simulink model "spectra_signals_new_2020b"  (R2020b)
settings: Solver=ode45  StartTime=0.0  StopTime=4.4  RelTol=1e-3  EnableMultiTasking=on
PreLoadFcn:
  | warning off all
undefined symbols (not defined in the file or in its folder): DiscIntNeverNeededParam
settings Model: Creator=morelos_zaragoza  LastModifiedBy=14083
settings DataIOCC: LimitDataPoints=on  SaveFormat=Array  SignalLoggingSaveFormat=ModelDataLogs  ReturnWorkspaceOutputs=off
settings OptimizationCC: ExpressionDepthLimit=2147483647  InitFltsAndDblsToZero=on  LifeSpan=inf
settings DebuggingCC: SaveWithParameterizedLinksMsg=none  UnderspecifiedInitializationDetection=Classic  MergeDetectMultiDrivingBlocksExec=none  SignalResolutionControl=TryResolveAllWithWarning  SolverPrmCheckMsg=warning  MultiTaskDSMMsg=warning  MultiTaskCondExecSysMsg=none  FcnCallInpInsideContextMsg=warning  StateNameClashWarn=warning  SFUnexpectedBacktrackingDiag=warning  SFNoUnconditionalDefaultTransitionDiag=warning  SFExecutionAtInitializationDiag=none  ArithmeticOperatorsInVariantConditions=warning
settings HardwareCC: ProdBitPerPointer=32  ProdBitPerSizeT=32  ProdBitPerPtrDiffT=32  ProdLargestAtomicFloat=None  ProdIntDivRoundTo=Undefined  ProdEndianess=Unspecified  ProdWordSize=32  ProdHWDeviceType=32-bit Generic
settings ModelReferenceCC: PropagateSignalLabelsOutOfModel=off
settings SFSimCC: SimUseLocalCustomCode=off  CustomCodeUndefinedFunction=UseInterfaceOnly
settings RTWCC: RTWUseLocalCustomCode=off
settings CodeAppCC: StateflowObjectComments=on
settings GRTTargetCC: TargetFcnLib=ansi_tfl_tmw.mat  TargetLangStandard=C89/C90 (ANSI)  CombineOutputUpdateFcns=off  GRTInterface=on
settings ConfigComp: CovMetricSettings=dw  CovSaveCumulativeToWorkspaceVar=on  CovSaveSingleToWorkspaceVar=on  CovExternalEMLEnable=off

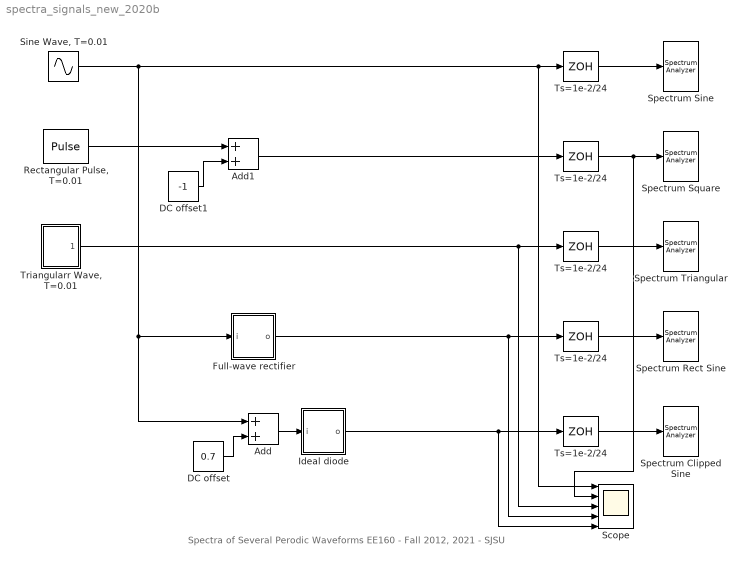
== system spectra_signals_new_2020b ==
  note: Spectra of Several Perodic Waveforms
      | EE160 - Fall 2012, 2021 - SJSU
  "     Ts=1e-2/24     " : ZeroOrderHold  SampleTime=1e-2/24
  "    Ts=1e-2/24    " : ZeroOrderHold  SampleTime=1e-2/24
  "  Ts=1e-2/24  " : ZeroOrderHold  SampleTime=1e-2/24
  " Ts=1e-2/24 " : ZeroOrderHold  SampleTime=1e-2/24
  Add : Sum
  Add1 : Sum
  DC offset : Constant  Value=0.7
  DC offset1 : Constant  Value=-1
  Full-wave rectifier : Subsystem  TreatAsAtomicUnit=on
  Ideal diode : Subsystem  TreatAsAtomicUnit=on
  "Rectangular Pulse, T=0.01" : DiscretePulseGenerator  Amplitude=2  Period=120  PulseWidth=120/3  SampleTime=1e-2/120
  Scope : Scope  NumInputPorts=5
  "Sine Wave, T=0.01" : Sin  Frequency=2*pi*100  SampleTime=0
  Spectrum Clipped Sine : SpectrumAnalyzer
  Spectrum Rect Sine : SpectrumAnalyzer
  Spectrum Sine : SpectrumAnalyzer
  Spectrum Square : SpectrumAnalyzer
  Spectrum Triangular : SpectrumAnalyzer
  "Triangularr Wave, T=0.01" : Subsystem  TreatAsAtomicUnit=on
  Ts=1e-2/24 : ZeroOrderHold  SampleTime=1e-2/24
  wires:
  Ts=1e-2/24/1 -> Spectrum Sine/1
  "Sine Wave, T=0.01"/1 -> Full-wave rectifier/1(i), Add/1, Ts=1e-2/24/1, Scope/1
  " Ts=1e-2/24 "/1 -> Spectrum Square/1, Scope/2
  "  Ts=1e-2/24  "/1 -> Spectrum Triangular/1
  "Triangularr Wave, T=0.01"/1(" ") -> "  Ts=1e-2/24  "/1, Scope/3
  "     Ts=1e-2/24     "/1 -> Spectrum Rect Sine/1
  Full-wave rectifier/1(o) -> "     Ts=1e-2/24     "/1, Scope/4
  Add/1 -> Ideal diode/1(i)
  DC offset/1 -> Add/2
  Ideal diode/1(o) -> "    Ts=1e-2/24    "/1, Scope/5
  "    Ts=1e-2/24    "/1 -> Spectrum Clipped Sine/1
  "Rectangular Pulse, T=0.01"/1 -> Add1/1
  DC offset1/1 -> Add1/2
  Add1/1 -> " Ts=1e-2/24 "/1

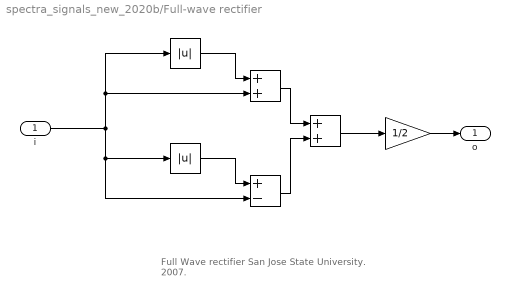
== system spectra_signals_new_2020b/Full-wave rectifier ==
  note: Full Wave rectifier
      | San Jose State University. 2007.
  i : Inport
  " " : Sum
  "   " : Sum  Inputs=+-
  "    " : Sum
  "        " : Gain  Gain=1/2
  "          " : Abs
  "                   " : Abs
  o : Outport
  wires:
  "                   "/1 -> " "/1
  "        "/1 -> o/1
  "          "/1 -> "   "/1
  " "/1 -> "    "/1
  "   "/1 -> "    "/2
  i/1 -> "                   "/1, " "/2, "          "/1, "   "/2
  "    "/1 -> "        "/1

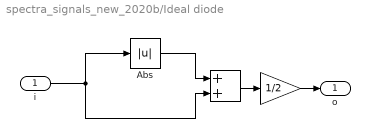
== system spectra_signals_new_2020b/Ideal diode ==
  i : Inport
  " " : Sum
  "        " : Gain  Gain=1/2
  Abs : Abs
  o : Outport
  wires:
  i/1 -> Abs/1, " "/2
  Abs/1 -> " "/1
  " "/1 -> "        "/1
  "        "/1 -> o/1

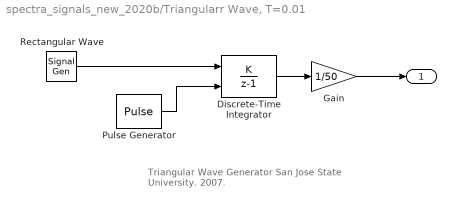
== system spectra_signals_new_2020b/Triangularr Wave, T=0.01 ==
  note: Triangular Wave Generator
      | San Jose State University. 2007.
  Discrete-Time Integrator : DiscreteIntegrator  IntegratorMethod=Accumulation: Forward Euler  ExternalReset=either  InitialCondition=50  SampleTime=1e-2/200  ICPrevOutput=DiscIntNeverNeededParam  ICPrevScaledInput=DiscIntNeverNeededParam
  Gain : Gain  Gain=1/50
  Pulse Generator : DiscretePulseGenerator  Amplitude=2  Period=480  PulseWidth=240  SampleTime=1e-2/240
  Rectangular Wave : SignalGenerator  WaveForm=square  Frequency=100
  " " : Outport
  wires:
  Discrete-Time Integrator/1 -> Gain/1
  Rectangular Wave/1 -> Discrete-Time Integrator/1
  Pulse Generator/1 -> Discrete-Time Integrator/2
  Gain/1 -> " "/1
